simulink model "test_05_cacc_sim"  (R2022b)
settings: Solver=VariableStepAuto  StartTime=0.0  StopTime=120  RelTol=1e-3
values from neighbouring files (symbols this model uses):
  accel = [1 0 1 0 -1 0 -0.5 0]    [cacc_test_01.m]    (also in test_01_cacc.m; test_02_cacc.m = [1 0 -1 0 -1 0 1 0]; test_04_cacc_hete.m = [traction_accel 0 bracking_accel 0 bracking_accel 0 traction; test_04_cacc_homo.m = [traction_accel 0 bracking_accel 0 bracking_accel 0 traction)
  dis_freq = 0.3    [test_04_cacc_hete.m]    (also in test_04_cacc_homo.m; test_05_cacc_hete.m = 4.5; test_05_cacc_homo.m = 4.5)
  e_init = [2 -1 -2]    [cacc_test_01.m]    (also in test_01_cacc.m; test_02_cacc.m; test_04_cacc_hete.m = [e_init1 e_init2 e_init3]; test_04_cacc_homo.m = [e_init1 e_init2 e_init3])
  h = 0.8    [cacc_test_01.m]    (also in test_01_cacc.m = 0.2; test_02_cacc.m; test_04_cacc_hete.m; test_04_cacc_homo.m)
  lv = 4.5    [test_04_cacc_hete.m]    (also in test_04_cacc_homo.m; test_05_cacc_hete.m; test_05_cacc_homo.m)
  p_init = [40 30 20 10]    [test_04_cacc_hete.m]    (also in test_04_cacc_homo.m; test_05_cacc_hete.m; test_05_cacc_homo.m)
  r = 8    [test_04_cacc_hete.m]    (also in test_04_cacc_homo.m; test_05_cacc_hete.m; test_05_cacc_homo.m)
  sim_mode = 1    [test_02_cacc.m]    (also in test_04_cacc_hete.m; test_04_cacc_homo.m; test_05_cacc_hete.m; test_05_cacc_homo.m)
  Ts = 0.02    [test_04_cacc_hete.m]    (also in test_04_cacc_homo.m; test_05_cacc_hete.m; test_05_cacc_homo.m)
  v_ref0 = 0    [cacc_test_01.m]    (also in test_01_cacc.m; test_02_cacc.m; test_04_cacc_hete.m = 5; test_04_cacc_homo.m = 5)
  wp = tril(ones(length(dt)))*dt    [cacc_test_01.m]    (also in test_01_cacc.m; test_02_cacc.m; test_04_cacc_hete.m; test_04_cacc_homo.m)
libraries: cstblocks x12, simulink x1
settings Model: Creator=phatdo  LastModifiedBy=phatdo
settings SolverCC: ZeroCrossAlgorithm=Adaptive
settings DataIOCC: ReturnWorkspaceOutputs=off
settings DebuggingCC: IgnoredZcDiagnostic=none

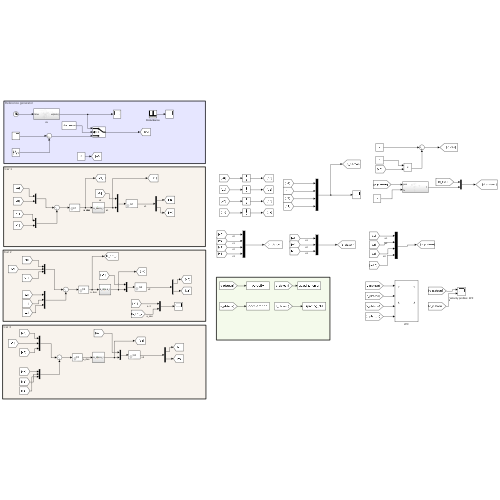
[thumbnail: Simulink's stored preview of the top-level diagram]
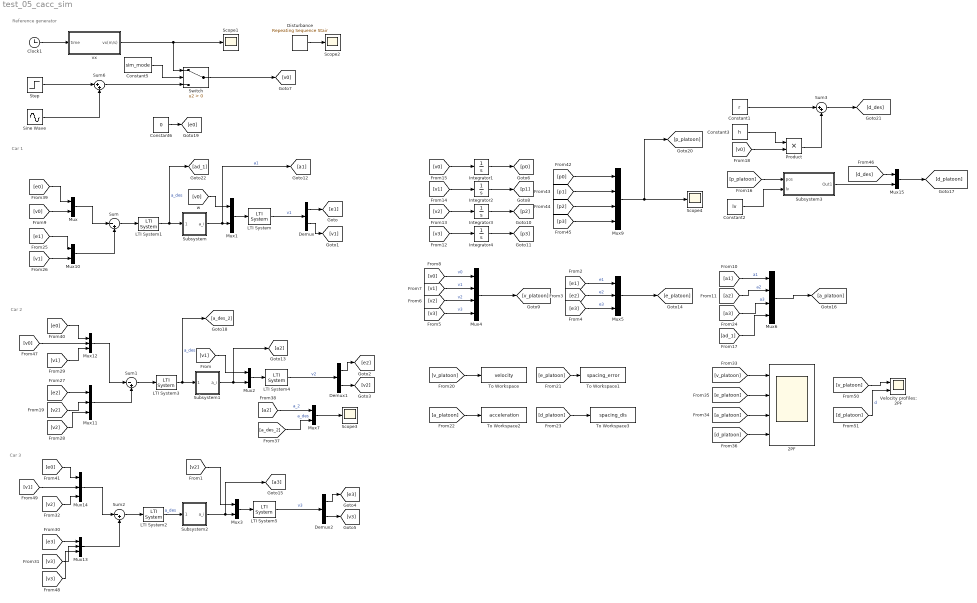
== system test_05_cacc_sim ==
  note: Car 3
  note: Car 2
  note: Car 1
  note: Reference generator
  2PF : Scope  NumInputPorts=4
  Clock1 : Clock
  Constant1 : Constant  Value=r
  Constant2 : Constant  Value=lv
  Constant3 : Constant  Value=h
  Constant5 : Constant  Value=sim_mode
  Constant6 : Constant  Value=0
  Demux : Demux  Outputs=2
  Demux1 : Demux  Outputs=2
  Demux2 : Demux  Outputs=2
  Disturbance : simulink/Sources/Repeating Sequence Stair  OutValues=[0 0 0 0 0 0 0 0 0 0.2 0 0 0 0 0 0 0 0].'  tsamp=5  OutMin=[]  OutMax=[]  OutDataTypeStr=double  OutputDataTypeScalingMode=double  OutDataType=fixdt(0,8)  ConRadixGroup=Best Precision: Vector-wise  OutScaling=2^-12
  Integrator1 : Integrator  InitialCondition=p_init(1)
  Integrator2 : Integrator  InitialCondition=p_init(2)
  Integrator3 : Integrator  InitialCondition=p_init(3)
  Integrator4 : Integrator  InitialCondition=p_init(4)
  LTI System : cstblocks/LTI System  sys=G1  IC=[e_init(1) 0]
  LTI System1 : cstblocks/LTI System  sys=K1  IC=[]
  LTI System2 : cstblocks/LTI System  sys=K3  IC=[]
  LTI System3 : cstblocks/LTI System  sys=K2  IC=[]
  LTI System4 : cstblocks/LTI System  sys=G2  IC=[e_init(2) 0]
  LTI System5 : cstblocks/LTI System  sys=G3  IC=[e_init(3) 0]
  Mux{,1..3,7,10,15} (7 alike) : Mux  Inputs=2
  Mux{5,11..14} (5 alike) : Mux  Inputs=3
  Mux4 : Mux
  Mux6 : Mux
  Mux9 : Mux
  Product : Product
  Scope{1..4} (4 alike) : Scope
  Sine Wave : Sin  Amplitude=5  Frequency=dis_freq  SampleTime=0
  Step : Step  Time=0  After=15  SampleTime=0
  Subsystem : Subsystem
  Subsystem1 : Subsystem
  Subsystem2 : Subsystem
  Subsystem3 : Subsystem
  Sum : Sum  Inputs=|-+
  Sum1 : Sum  Inputs=|-+
  Sum2 : Sum  Inputs=|-+
  Sum3 : Sum  Inputs=|++
  Sum6 : Sum  Inputs=|++
  Switch : Switch  Criteria=u2 > Threshold  SaturateOnIntegerOverflow=off  InputSameDT=off
  To Workspace : ToWorkspace  VariableName=velocity  SaveFormat=Timeseries  SampleTime=-1
  To Workspace1 : ToWorkspace  VariableName=spacing_error  SaveFormat=Timeseries  SampleTime=-1
  To Workspace2 : ToWorkspace  VariableName=acceleration  SaveFormat=Timeseries  SampleTime=-1
  To Workspace3 : ToWorkspace  VariableName=spacing_dis  SaveFormat=Timeseries  SampleTime=-1
  Velocity profiles: 2PF : Scope  NumInputPorts=2
  vx : Subsystem
  wires:
  Sum/1 -> LTI System1/1
  Sum1/1 -> LTI System3/1
  Sum2/1 -> LTI System2/1
  LTI System4/1 -> Demux1/1  "v2"
  LTI System5/1 -> Demux2/1  "v3"
  Mux1/1 -> LTI System/1
  LTI System1/1 -> Subsystem/1(a_des), [ad_1]  "a_des"
  Mux2/1 -> LTI System4/1
  Mux3/1 -> LTI System5/1
  LTI System3/1 -> Subsystem1/1(a_des), [a_des_2]  "a_des"
  LTI System/1 -> Demux/1  "v1"
  [e0] -> Mux/1
  Demux/1 -> [e1]
  Demux/2 -> [v1]
  [v1] -> Mux2/1
  Demux1/1 -> [e2]
  Demux1/2 -> [v2]
  Demux2/1 -> [e3]
  Demux2/2 -> [v3]
  [v2] -> Mux3/1
  [v0] -> Mux4/1  "v0"
  [v1] -> Mux4/2  "v1"
  [v2] -> Mux4/3  "v2"
  [v3] -> Mux4/4  "v3"
  [e1] -> Mux5/1  "e1"
  [e2] -> Mux5/2  "e2"
  [e3] -> Mux5/3  "e3"
  [v0] -> Mux1/1
  [v0] -> Mux/2
  [v0] -> Integrator1/1
  [v1] -> Integrator2/1
  [v2] -> Integrator3/1
  [v3] -> Integrator4/1
  Integrator1/1 -> [p0]
  Integrator2/1 -> [p1]
  Integrator3/1 -> [p2]
  Integrator4/1 -> [p3]
  LTI System2/1 -> Subsystem2/1(a_des)  "a_des"
  [a1] -> Mux6/1  "a1"
  [a2] -> Mux6/2  "a2"
  [a3] -> Mux6/3  "a3"
  Clock1/1 -> vx/1(time)
  vx/1(vx(m/s)) -> Scope1/1, Switch/1
  [v1] -> Mux10/2
  Mux10/1 -> Sum/2
  Mux/1 -> Sum/1
  [e0] -> Mux12/1
  Mux12/1 -> Sum1/1
  [v1] -> Mux12/3
  [e2] -> Mux11/1
  [v2] -> Mux11/3
  Mux11/1 -> Sum1/2
  [e3] -> Mux13/1
  [v3] -> Mux13/2
  Mux13/1 -> Sum2/2
  [e0] -> Mux14/1
  Mux14/1 -> Sum2/1
  Step/1 -> Sum6/1
  Sine Wave/1 -> Sum6/2
  Constant5/1 -> Switch/2
  Switch/1 -> [v0]
  Sum6/1 -> Switch/3
  Mux4/1 -> [v_platoon]
  Mux5/1 -> [e_platoon]
  Mux6/1 -> [a_platoon]
  [v_platoon] -> To Workspace/1
  [e_platoon] -> To Workspace1/1
  [a_platoon] -> To Workspace2/1
  [d_platoon] -> To Workspace3/1
  [e_platoon] -> 2PF/2
  [v_platoon] -> 2PF/1
  [a_platoon] -> 2PF/3
  Disturbance/1 -> Scope2/1
  [e1] -> Mux10/1
  [a2] -> Mux7/1  "a_2"
  [a_des_2] -> Mux7/2  "a_des"
  Mux7/1 -> Scope3/1
  Constant6/1 -> [e0]
  [p1] -> Mux9/2
  [p2] -> Mux9/3
  [p3] -> Mux9/4
  Mux9/1 -> [p_platoon], Scope4/1
  [p0] -> Mux9/1
  Constant2/1 -> Subsystem3/2(lv)
  [p_platoon] -> Subsystem3/1(pos)
  Constant1/1 -> Sum3/1
  Constant3/1 -> Product/1
  [v0] -> Product/2
  Product/1 -> Sum3/2
  Sum3/1 -> [d_des]
  [d_platoon] -> 2PF/4
  Subsystem3/1(Out1) -> Mux15/2
  [d_des] -> Mux15/1
  Mux15/1 -> [d_platoon]
  [ad_1] -> Mux6/4
  [v2] -> Mux11/2
  [v0] -> Mux12/2
  [v3] -> Mux13/3
  [v2] -> Mux14/3
  [v1] -> Mux14/2
  [v_platoon] -> Velocity profiles: 2PF/1
  [d_platoon] -> Velocity profiles: 2PF/2  "d"
  Subsystem/1(a_i) -> [a1], Mux1/2  "a1"
  Subsystem1/1(a_i) -> [a2], Mux2/2
  Subsystem2/1(a_i) -> [a3], Mux3/2

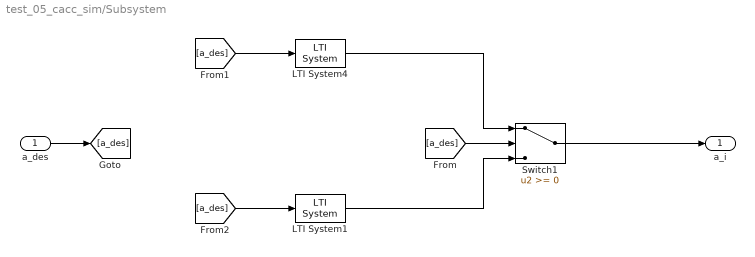
== system test_05_cacc_sim/Subsystem ==
  a_des : Inport
  LTI System1 : cstblocks/LTI System  sys=Ge_b_1  IC=[]
  LTI System4 : cstblocks/LTI System  sys=Ge_a_1  IC=[]
  Switch1 : Switch  SaturateOnIntegerOverflow=off  InputSameDT=off
  a_i : Outport
  wires:
  a_des/1 -> [a_des]
  [a_des] -> Switch1/2
  Switch1/1 -> a_i/1
  LTI System4/1 -> Switch1/1
  LTI System1/1 -> Switch1/3
  [a_des] -> LTI System4/1
  [a_des] -> LTI System1/1

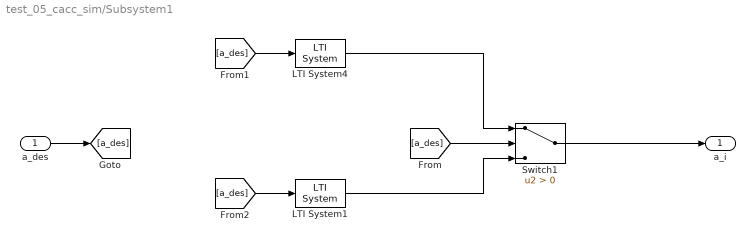
== system test_05_cacc_sim/Subsystem1 ==
  a_des : Inport
  LTI System1 : cstblocks/LTI System  sys=Ge_b_2  IC=[]
  LTI System4 : cstblocks/LTI System  sys=Ge_a_2  IC=[]
  Switch1 : Switch  Criteria=u2 > Threshold  SaturateOnIntegerOverflow=off  InputSameDT=off
  a_i : Outport
  wires:
  a_des/1 -> [a_des]
  [a_des] -> Switch1/2
  Switch1/1 -> a_i/1
  LTI System4/1 -> Switch1/1
  LTI System1/1 -> Switch1/3
  [a_des] -> LTI System4/1
  [a_des] -> LTI System1/1

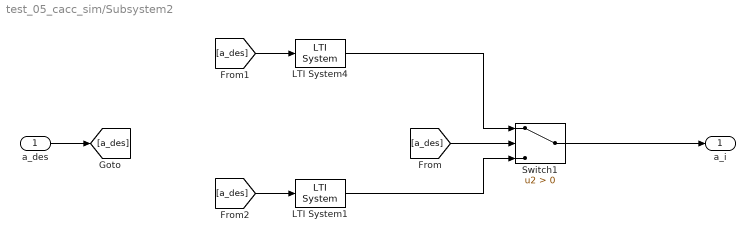
== system test_05_cacc_sim/Subsystem2 ==
  a_des : Inport
  LTI System1 : cstblocks/LTI System  sys=Ge_b_3  IC=[]
  LTI System4 : cstblocks/LTI System  sys=Ge_a_3  IC=[]
  Switch1 : Switch  Criteria=u2 > Threshold  SaturateOnIntegerOverflow=off  InputSameDT=off
  a_i : Outport
  wires:
  a_des/1 -> [a_des]
  [a_des] -> Switch1/2
  Switch1/1 -> a_i/1
  LTI System4/1 -> Switch1/1
  LTI System1/1 -> Switch1/3
  [a_des] -> LTI System4/1
  [a_des] -> LTI System1/1

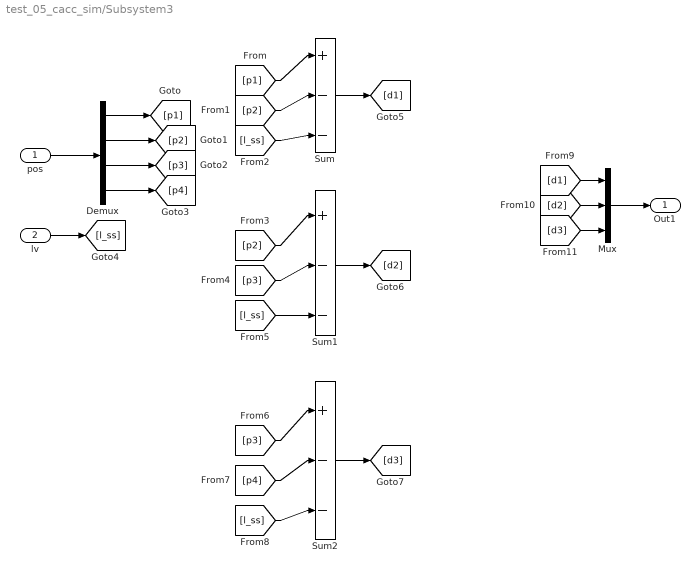
== system test_05_cacc_sim/Subsystem3 ==
  pos : Inport
  lv : Inport  Port=2
  Demux : Demux
  Mux : Mux  Inputs=3
  Sum : Sum  Inputs=|+--
  Sum1 : Sum  Inputs=|+--
  Sum2 : Sum  Inputs=|+--
  Out1 : Outport
  wires:
  pos/1 -> Demux/1
  Demux/1 -> [p1]
  Demux/2 -> [p2]
  Demux/3 -> [p3]
  Demux/4 -> [p4]
  [p1] -> Sum/1
  [p2] -> Sum/2
  lv/1 -> [l_ss]
  [l_ss] -> Sum/3
  Sum/1 -> [d1]
  [p3] -> Sum1/2
  Sum1/1 -> [d2]
  [p2] -> Sum1/1
  [l_ss] -> Sum1/3
  [l_ss] -> Sum2/3
  [p4] -> Sum2/2
  [p3] -> Sum2/1
  Sum2/1 -> [d3]
  [d1] -> Mux/1
  [d2] -> Mux/2
  [d3] -> Mux/3
  Mux/1 -> Out1/1

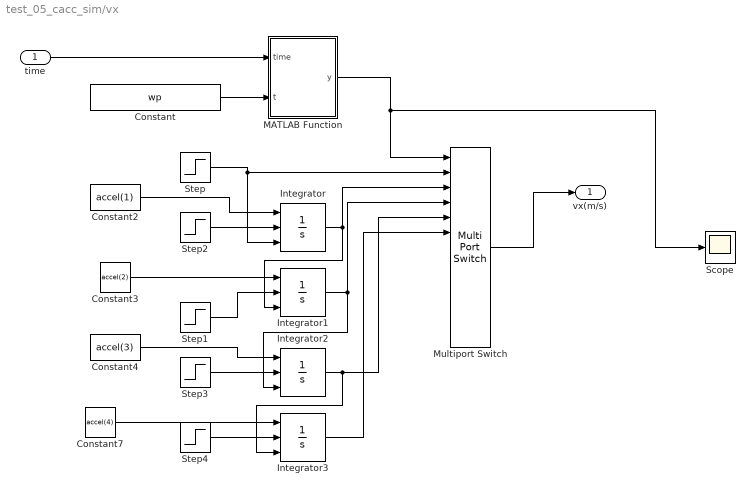
== system test_05_cacc_sim/vx ==
  time : Inport  SampleTime=Ts
  Constant : Constant  Value=wp
  Constant2 : Constant  Value=accel(1)
  Constant3 : Constant  Value=accel(2)
  Constant4 : Constant  Value=accel(3)
  Constant7 : Constant  Value=accel(4)
  Integrator{,1..3} (4 alike) : Integrator  ExternalReset=rising  InitialConditionSource=external
  MATLAB Function : MATLAB Function  TreatAsAtomicUnit=on
  Multiport Switch : MultiPortSwitch  Inputs=12  SaturateOnIntegerOverflow=off  InputSameDT=off
  Scope : Scope
  Step : Step  Time=0  Before=v_ref0  After=v_ref0  SampleTime=0
  Step1 : Step  Time=wp(2)  SampleTime=0
  Step2 : Step  Time=wp(1)  SampleTime=0
  Step3 : Step  Time=wp(3)  SampleTime=0
  Step4 : Step  Time=wp(4)  SampleTime=0
  vx(m/s) : Outport
  wires:
  Step/1 -> Integrator/3, Multiport Switch/2
  Constant/1 -> MATLAB Function/2(t)
  Constant2/1 -> Integrator/1
  Multiport Switch/1 -> vx(m/s)/1
  Integrator/1 -> Integrator1/3, Multiport Switch/3
  Step2/1 -> Integrator/2
  Constant3/1 -> Integrator1/1
  Integrator1/1 -> Integrator2/3, Multiport Switch/4
  Step1/1 -> Integrator1/2
  time/1 -> MATLAB Function/1(time)
  Step3/1 -> Integrator2/2
  Constant4/1 -> Integrator2/1
  Integrator2/1 -> Integrator3/3, Multiport Switch/5
  Integrator3/1 -> Multiport Switch/6
  Step4/1 -> Integrator3/2
  Constant7/1 -> Integrator3/1
  MATLAB Function/1(y) -> Scope/1, Multiport Switch/1

== matlab function test_05_cacc_sim/vx/MATLAB Function ==
  data: time input; t input; y output
function y = fcn(time,t)
t1 = t(1);
t2 = t(2);
t3 = t(3);
t4 = t(4);
% t5 = t(5);
% t6 = t(6);
% t7 = t(7);
% t8 = t(8);

if time<=t1
    y = 1;
elseif time>t1 && time <= t2
    y = 2;
elseif time>t2 && time <= t3
    y = 3;
elseif time>t3 && time <= t4
    y = 4;
% elseif time>t4 && time <= t5
%     y = 5;
% elseif time>t5 && time <= t6
%     y = 6;
% elseif time>t6 && time <= t7
%     y = 7;
% elseif time>t7 && time <= t8
%     y = 8;
else 
%     y = 9;
    y = 5;
end
